simulink model "full_car_model"  (Simulink 7.0)
settings: Solver=ode45  StartTime=0.0  StopTime=120  RelTol=1e-3
undefined symbols (not defined in the file): a, b, c, c01, c02, c03, c04, c1, c2, c3, c4, d, Ix, Iy, k01, k02, k03, k04, k1, k2, k3, k4, M, m1, m2, m3, m4, sigbuilder_block
(part 1 of 2)
settings Model: Creator=Svitlana i Oleksandr  LastModifiedBy=Svitlana i Oleksandr
settings DataIOCC: LimitDataPoints=off

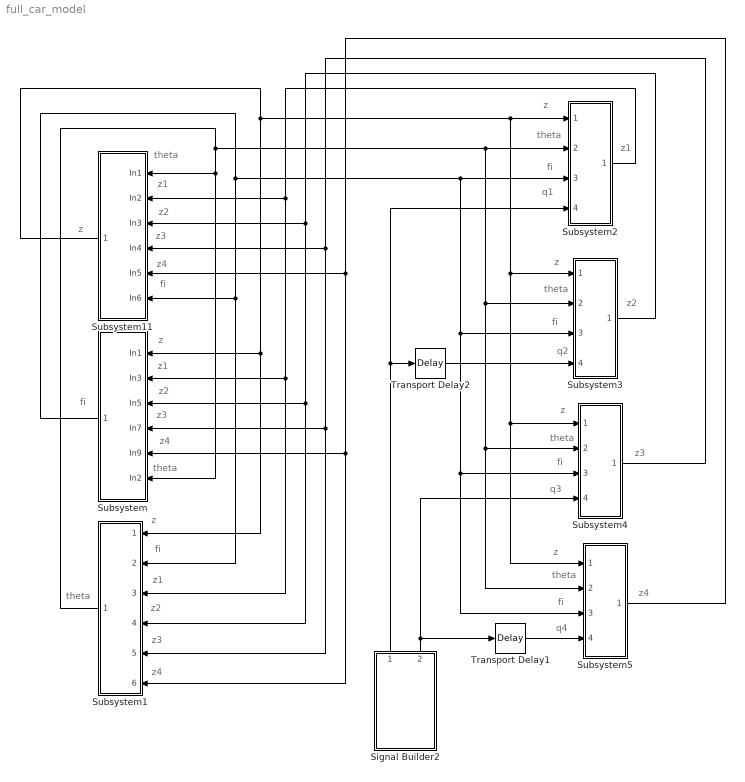
== system full_car_model ==
  note: z
  note: theta
  note: z1
  note: z2
  note: z3
  note: z4
  note: fi
  note: fi
  note: z
  note: z1
  note: z2
  note: z3
  note: z4
  note: theta
  note: theta
  note: z
  note: fi
  note: z1
  note: z2
  note: z3
  note: z4
  note: z1
  note: z
  note: theta
  note: fi
  note: q1
  note: z2
  note: z
  note: theta
  note: fi
  note: q2
  note: z3
  note: z
  note: theta
  note: fi
  note: q3
  note: z4
  note: q4
  note: z
  note: theta
  note: fi
  Signal Builder2 : Subsystem  Tag=STV Subsys  Orientation=up  LoadFcn=sigbuilder_block('load');  StartFcn=sigbuilder_block('start');  StopFcn=sigbuilder_block('stop');  ClipboardFcn=sigbuilder_block('clipboard');  mask(Sigbuilder block){}
      mask help: Sigbuilder GUI
      mask init:
      | if ~strcmp(get_param(bdroot(gcbh),'SimulationStatus'),'stopped') tuvar = sigbuilder_block('maskInit'); end
      settings: CopyFcn=sigbuilder_block('copy');  DeleteFcn=sigbuilder_block('delete');  ModelCloseFcn=sigbuilder_block('modelClose');  PreSaveFcn=sigbuilder_block('preSave');  NameChangeFcn=sigbuilder_block('namechange');  OpenFcn=sigbuilder_block('open',[124.5 96 550.5 363.75 ]);  CloseFcn=sigbuilder_block('close');
      mask Display: plot(0,0,100,100,[10,10,40,40,10],[80,20,20,80,80],[40,10],[50,50], [40,27,10],[65,72,56],[40,25,25,10],[28,28,43,43]);
  Subsystem : Subsystem  Orientation=left
  Subsystem1 : Subsystem  Orientation=left
  Subsystem11 : Subsystem  Orientation=left
  Subsystem2 : Subsystem
  Subsystem3 : Subsystem
  Subsystem4 : Subsystem
  Subsystem5 : Subsystem
  Transport Delay1 : TransportDelay  DelayTime=0.2
  Transport Delay2 : TransportDelay  DelayTime=0.2
  wires:
  Subsystem11/1(Out1) -> Subsystem/1(In1), Subsystem1/1(In1), Subsystem2/1(In1), Subsystem3/1(In1), Subsystem4/1(In1), Subsystem5/1(In1)
  Subsystem/1(Out1) -> Subsystem11/6(In6), Subsystem1/2(In2), Subsystem2/3(In3), Subsystem3/3(In3), Subsystem4/3(In3), Subsystem5/3(In3)
  Subsystem1/1(Out1) -> Subsystem11/1(In1), Subsystem/6(In2), Subsystem2/2(In2), Subsystem3/2(In2), Subsystem4/2(In2), Subsystem5/2(In2)
  Subsystem2/1(Out1) -> Subsystem11/2(In2), Subsystem/2(In3), Subsystem1/3(In3)
  Subsystem3/1(Out1) -> Subsystem11/3(In3), Subsystem/3(In5), Subsystem1/4(In6)
  Transport Delay2/1 -> Subsystem3/4(In4)
  Subsystem4/1(Out1) -> Subsystem11/4(In4), Subsystem/4(In7), Subsystem1/5(In9)
  Subsystem5/1(Out1) -> Subsystem11/5(In5), Subsystem/5(In9), Subsystem1/6(In12)
  Transport Delay1/1 -> Subsystem5/4(In7)
  Signal Builder2/2(Signal 2) -> Transport Delay1/1, Subsystem4/4(In4)
  Signal Builder2/1(Signal 1) -> Subsystem2/4(In4), Transport Delay2/1

== system full_car_model/Signal Builder2 ==
  Demux : Demux  Tag=STV Demux  Outputs=2
  FromWs : FromWorkspace  Tag=STV FromWs  VariableName=tuvar  SampleTime=0  SigBuilderData=DataTag0  VnvData=DataTag1
      SigBuilderData=|
      | channels(1).label = 'Signal 1'
      | channels(1).allXData = {[0 4 4 6 6 10]}
      | channels(1).allYData = {[0 0 0.1 0.1 0 0]}
      | channels(2).label = 'Signal 2'
      | channels(2).allXData = {[0 10]}
      | channels(2).allYData = {[0 0]}
      | common.afterFinalStr = 'Extrapolate'
      | common.sampleTime = 0
      | dataSet.timeRange = [0 10]
      | dataSet.name = 'Group 1'
  Signal 1 : Outport  Tag=STV Outport  OutDataType=sfix(16)  OutScaling=2^0
  Signal 2 : Outport  Tag=STV Outport  Port=2
  wires:
  FromWs/1 -> Demux/1
  Demux/1 -> Signal 1/1
  Demux/2 -> Signal 2/1

== system full_car_model/Subsystem ==
  note: fi
  note: z
  note: theta
  note: fi
  note: z1
  note: k1
  note: c1
  note: k2
  note: c2
  note: z
  note: theta
  note: fi
  note: z2
  note: k3
  note: c3
  note: z
  note: theta
  note: fi
  note: z3
  note: k4
  note: c4
  note: z
  note: theta
  note: fi
  note: z4
  note: fi
  note: theta
  note: z
  In1 : Inport  Orientation=left
  In3 : Inport  Orientation=left  Port=2
  In5 : Inport  Orientation=left  Port=3
  In7 : Inport  Orientation=left  Port=4
  In9 : Inport  Orientation=left  Port=5
  In2 : Inport  Orientation=left  Port=6
  Gain2 : Gain  Gain=1/Ix  ParameterDataType=sfix(16)  ParameterScaling=2^0  OutDataType=sfix(16)  OutScaling=2^0
  Integrator3 : Integrator
  Integrator4 : Integrator
  Subsystem3 : Subsystem  Orientation=left
  Subsystem4 : Subsystem  Orientation=left
  Subsystem5 : Subsystem  Orientation=left
  Subsystem6 : Subsystem  Orientation=left
  Sum2 : Sum  Inputs=----++++  OutDataType=sfix(16)  OutScaling=2^0
  Out1 : Outport
  wires:
  Sum2/1 -> Gain2/1
  Gain2/1 -> Integrator3/1
  Integrator3/1 -> Integrator4/1
  Integrator4/1 -> Subsystem3/3(In3), Subsystem4/3(In3), Subsystem5/3(In3), Subsystem6/3(In3), Out1/1
  Subsystem3/1(Out1) -> Sum2/1
  Subsystem3/2(Out2) -> Sum2/2
  Subsystem4/1(Out1) -> Sum2/3
  Subsystem4/2(Out2) -> Sum2/4
  Subsystem5/1(Out1) -> Sum2/5
  Subsystem5/2(Out2) -> Sum2/6
  Subsystem6/1(Out1) -> Sum2/7
  Subsystem6/2(Out2) -> Sum2/8
  In3/1 -> Subsystem3/4(In4)
  In5/1 -> Subsystem4/4(In4)
  In7/1 -> Subsystem5/4(In4)
  In9/1 -> Subsystem6/4(In4)
  In1/1 -> Subsystem3/1(In1), Subsystem4/1(In1), Subsystem5/1(In1), Subsystem6/1(In1)
  In2/1 -> Subsystem3/2(In2), Subsystem4/2(In2), Subsystem5/2(In2), Subsystem6/2(In2)

== system full_car_model/Subsystem1 ==
  note: theta
  note: k1
  note: c1
  note: z
  note: theta
  note: fi
  note: z1
  note: k2
  note: c2
  note: z
  note: theta
  note: fi
  note: z2
  note: k3
  note: c3
  note: z
  note: theta
  note: fi
  note: z3
  note: k4
  note: c4
  note: z
  note: fi
  note: z
  note: theta
  note: fi
  note: z4
  In1 : Inport  Orientation=left
  In2 : Inport  Orientation=left  Port=2
  In3 : Inport  Orientation=left  Port=3
  In6 : Inport  Orientation=left  Port=4
  In9 : Inport  Orientation=left  Port=5
  In12 : Inport  Orientation=left  Port=6
  Gain3 : Gain  Gain=1/Iy  ParameterDataType=sfix(16)  ParameterScaling=2^0  OutDataType=sfix(16)  OutScaling=2^0
  Integrator5 : Integrator
  Integrator6 : Integrator
  Subsystem10 : Subsystem  Orientation=left
  Subsystem7 : Subsystem  Orientation=left
  Subsystem8 : Subsystem  Orientation=left
  Subsystem9 : Subsystem  Orientation=left
  Sum3 : Sum  Inputs=++--++--  OutDataType=sfix(16)  OutScaling=2^0
  Out1 : Outport
  wires:
  Sum3/1 -> Gain3/1
  Gain3/1 -> Integrator5/1
  Integrator5/1 -> Integrator6/1
  Subsystem7/1(Out1) -> Sum3/1
  Subsystem7/2(Out2) -> Sum3/2
  Subsystem8/1(Out1) -> Sum3/3
  Subsystem8/2(Out2) -> Sum3/4
  Subsystem9/1(Out1) -> Sum3/5
  Subsystem9/2(Out2) -> Sum3/6
  Subsystem10/1(Out1) -> Sum3/7
  Subsystem10/2(Out2) -> Sum3/8
  Integrator6/1 -> Subsystem7/2(In2), Subsystem8/2(In2), Subsystem9/2(In2), Subsystem10/2(In2), Out1/1
  In3/1 -> Subsystem7/4(In4)
  In6/1 -> Subsystem8/4(In4)
  In9/1 -> Subsystem9/4(In4)
  In12/1 -> Subsystem10/4(In4)
  In1/1 -> Subsystem7/1(In1), Subsystem8/1(In1), Subsystem9/1(In1), Subsystem10/1(In1)
  In2/1 -> Subsystem7/3(In3), Subsystem8/3(In3), Subsystem9/3(In3), Subsystem10/3(In3)

== system full_car_model/Subsystem11 ==
  note: z
  note: z
  note: theta
  note: fi
  note: z1
  note: k1
  note: c1
  note: z
  note: theta
  note: fi
  note: z2
  note: k2
  note: c2
  note: z
  note: theta
  note: fi
  note: z3
  note: k3
  note: c3
  note: z
  note: theta
  note: fi
  note: z4
  note: z
  note: theta
  note: k4
  note: c4
  note: fi
  In1 : Inport  Orientation=left  OutDataType=sfix(16)  OutScaling=2^0
  In2 : Inport  Orientation=left  Port=2  OutDataType=sfix(16)  OutScaling=2^0
  In3 : Inport  Orientation=left  Port=3  OutDataType=sfix(16)  OutScaling=2^0
  In4 : Inport  Orientation=left  Port=4  OutDataType=sfix(16)  OutScaling=2^0
  In5 : Inport  Orientation=left  Port=5  OutDataType=sfix(16)  OutScaling=2^0
  In6 : Inport  Orientation=left  Port=6  OutDataType=sfix(16)  OutScaling=2^0
  Gain1 : Gain  Gain=1/M  ParameterDataType=sfix(16)  ParameterScaling=2^0  OutDataType=sfix(16)  OutScaling=2^0
  Integrator1 : Integrator
  Integrator2 : Integrator
  Subsystem : Subsystem  Orientation=left
  Subsystem1 : Subsystem  Orientation=left
  Subsystem2 : Subsystem  Orientation=left
  Subsystem40 : Subsystem  Orientation=left
  Sum1 : Sum  Inputs=--------  OutDataType=sfix(16)  OutScaling=2^0
  Out1 : Outport  OutDataType=sfix(16)  OutScaling=2^0
  wires:
  Sum1/1 -> Gain1/1
  Gain1/1 -> Integrator1/1
  Integrator1/1 -> Integrator2/1
  Subsystem40/1(Out1) -> Sum1/8
  Subsystem40/2(Out2) -> Sum1/7
  Subsystem/1(Out1) -> Sum1/6
  Subsystem/2(Out2) -> Sum1/5
  In2/1 -> Subsystem40/4(In4)
  In3/1 -> Subsystem/4(In4)
  In4/1 -> Subsystem1/4(In4)
  In5/1 -> Subsystem2/4(In4)
  Integrator2/1 -> Out1/1, Subsystem40/1(In1), Subsystem/1(In1), Subsystem1/1(In1), Subsystem2/1(In1)
  Subsystem1/1(Out1) -> Sum1/4
  Subsystem1/2(Out2) -> Sum1/3
  Subsystem2/1(Out1) -> Sum1/2
  Subsystem2/2(Out2) -> Sum1/1
  In1/1 -> Subsystem40/2(In2), Subsystem/2(In2), Subsystem1/2(In2), Subsystem2/2(In2)
  In6/1 -> Subsystem40/3(In3), Subsystem/3(In3), Subsystem1/3(In3), Subsystem2/3(In3)

== system full_car_model/Subsystem2 ==
  note: z1
  note: k1
  note: z
  note: theta
  note: fi
  note: z1
  note: c1
  note: z
  note: theta
  note: fi
  note: z1
  note: k01
  note: z1
  note: q1
  note: c01
  note: z1
  note: q1
  note: z
  note: theta
  note: fi
  note: q1
  In1 : Inport  Orientation=left
  In2 : Inport  Orientation=left  Port=2
  In3 : Inport  Orientation=left  Port=3
  In4 : Inport  Orientation=left  Port=4
  Gain4 : Gain  Gain=1/m1  ParameterDataType=sfix(16)  ParameterScaling=2^0  OutDataType=sfix(16)  OutScaling=2^0
  Integrator7 : Integrator
  Integrator8 : Integrator
  Subsystem24 : Subsystem  Orientation=left
  Subsystem25 : Subsystem  Orientation=left
  Subsystem26 : Subsystem  Orientation=left
  Subsystem27 : Subsystem  Orientation=left
  Sum8 : Sum  Inputs=++--  OutDataType=sfix(16)  OutScaling=2^0
  Out1 : Outport  OutDataType=sfix(16)  OutScaling=2^0
  wires:
  Gain4/1 -> Integrator7/1
  Integrator7/1 -> Integrator8/1
  Sum8/1 -> Gain4/1
  Subsystem24/1(Out2) -> Sum8/1
  Subsystem25/1(Out2) -> Sum8/2
  Subsystem26/1(Out2) -> Sum8/3
  Subsystem27/1(Out2) -> Sum8/4
  In1/1 -> Subsystem24/1(In1), Subsystem25/1(In1)
  In2/1 -> Subsystem24/2(In3), Subsystem25/2(In3)
  In3/1 -> Subsystem24/3(In4), Subsystem25/3(In4)
  Integrator8/1 -> Out1/1, Subsystem24/4(In5), Subsystem25/4(In5), Subsystem26/1(In1), Subsystem27/1(In1)
  In4/1 -> Subsystem26/2(In5), Subsystem27/2(In5)

== system full_car_model/Subsystem3 ==
  note: z2
  note: k2
  note: z
  note: theta
  note: fi
  note: z2
  note: c2
  note: z
  note: theta
  note: fi
  note: z2
  note: k02
  note: z2
  note: q2
  note: c02
  note: z2
  note: q2
  note: z
  note: fi
  note: q2
  In1 : Inport  Orientation=left
  In2 : Inport  Orientation=left  Port=2
  In3 : Inport  Orientation=left  Port=3
  In4 : Inport  Orientation=left  Port=4
  Gain5 : Gain  Gain=1/m2  ParameterDataType=sfix(16)  ParameterScaling=2^0  OutDataType=sfix(16)  OutScaling=2^0
  Integrator10 : Integrator
  Integrator9 : Integrator
  Subsystem28 : Subsystem  Orientation=left
  Subsystem29 : Subsystem  Orientation=left
  Subsystem30 : Subsystem  Orientation=left
  Subsystem31 : Subsystem  Orientation=left
  Sum5 : Sum  Inputs=++--  OutDataType=sfix(16)  OutScaling=2^0
  Out1 : Outport  OutDataType=sfix(16)  OutScaling=2^0
  wires:
  Sum5/1 -> Gain5/1
  Gain5/1 -> Integrator9/1
  Integrator9/1 -> Integrator10/1
  Subsystem28/1(Out2) -> Sum5/1
  Subsystem29/1(Out2) -> Sum5/2
  Subsystem30/1(Out2) -> Sum5/3
  Subsystem31/1(Out2) -> Sum5/4
  In1/1 -> Subsystem28/1(In1), Subsystem29/1(In1)
  In2/1 -> Subsystem28/2(In3), Subsystem29/2(In3)
  In3/1 -> Subsystem28/3(In4), Subsystem29/3(In4)
  Integrator10/1 -> Out1/1, Subsystem28/4(In5), Subsystem29/4(In5), Subsystem30/1(In1), Subsystem31/1(In1)
  In4/1 -> Subsystem30/2(In5), Subsystem31/2(In5)

== system full_car_model/Subsystem4 ==
  note: z3
  note: c3
  note: z
  note: theta
  note: fi
  note: z3
  note: k3
  note: z
  note: theta
  note: fi
  note: z3
  note: k03
  note: z3
  note: q3
  note: c03
  note: z3
  note: q3
  note: z
  note: theta
  note: fi
  note: q3
  In1 : Inport  Orientation=left
  In2 : Inport  Orientation=left  Port=2
  In3 : Inport  Orientation=left  Port=3
  In4 : Inport  Orientation=left  Port=4
  Gain6 : Gain  Gain=1/m3  ParameterDataType=sfix(16)  ParameterScaling=2^0  OutDataType=sfix(16)  OutScaling=2^0
  Integrator11 : Integrator
  Integrator12 : Integrator
  Subsystem32 : Subsystem  Orientation=left
  Subsystem33 : Subsystem  Orientation=left
  Subsystem34 : Subsystem  Orientation=left
  Subsystem35 : Subsystem  Orientation=left
  Sum6 : Sum  Inputs=++--  OutDataType=sfix(16)  OutScaling=2^0
  Out1 : Outport  OutDataType=sfix(16)  OutScaling=2^0
  wires:
  Sum6/1 -> Gain6/1
  Gain6/1 -> Integrator12/1
  Integrator12/1 -> Integrator11/1
  Subsystem32/1(Out2) -> Sum6/1
  Subsystem33/1(Out2) -> Sum6/2
  Subsystem34/1(Out2) -> Sum6/3
  Subsystem35/1(Out2) -> Sum6/4
  In1/1 -> Subsystem32/1(In1), Subsystem33/1(In1)
  In2/1 -> Subsystem32/2(In3), Subsystem33/2(In3)
  In3/1 -> Subsystem32/3(In4), Subsystem33/3(In4)
  Integrator11/1 -> Out1/1, Subsystem32/4(In5), Subsystem33/4(In5), Subsystem34/1(In1), Subsystem35/1(In1)
  In4/1 -> Subsystem34/2(In5), Subsystem35/2(In5)

== system full_car_model/Subsystem5 ==
  note: z4
  note: k4
  note: z
  note: theta
  note: fi
  note: z4
  note: c4
  note: z
  note: theta
  note: fi
  note: z4
  note: k04
  note: z4
  note: q4
  note: c04
  note: z4
  note: q4
  note: z
  note: theta
  note: fi
  note: z4
  note: q4
  In1 : Inport  Orientation=left
  In2 : Inport  Orientation=left  Port=2
  In3 : Inport  Orientation=left  Port=3
  In7 : Inport  Orientation=left  Port=4
  Gain7 : Gain  Gain=1/m4  ParameterDataType=sfix(16)  ParameterScaling=2^0  OutDataType=sfix(16)  OutScaling=2^0
  Integrator13 : Integrator
  Integrator14 : Integrator
  Subsystem36 : Subsystem  Orientation=left
  Subsystem37 : Subsystem  Orientation=left
  Subsystem38 : Subsystem  Orientation=left
  Subsystem39 : Subsystem  Orientation=left
  Sum7 : Sum  Inputs=++--  OutDataType=sfix(16)  OutScaling=2^0
  Out1 : Outport  OutDataType=sfix(16)  OutScaling=2^0
  wires:
  Sum7/1 -> Gain7/1
  Gain7/1 -> Integrator14/1
  Integrator14/1 -> Integrator13/1
  Subsystem36/1(Out2) -> Sum7/1
  Subsystem37/1(Out2) -> Sum7/2
  Subsystem38/1(Out2) -> Sum7/3
  Subsystem39/1(Out2) -> Sum7/4
  In1/1 -> Subsystem36/1(In1), Subsystem37/1(In1)
  In2/1 -> Subsystem36/2(In3), Subsystem37/2(In3)
  In3/1 -> Subsystem36/3(In4), Subsystem37/3(In4)
  In7/1 -> Subsystem38/2(In5), Subsystem39/2(In5)
  Integrator13/1 -> Out1/1, Subsystem36/4(In5), Subsystem37/4(In5), Subsystem38/1(In1), Subsystem39/1(In1)

== system full_car_model/Subsystem/Subsystem3 ==
  note: z
  note: k1
  note: theta
  note: fi
  note: z1
  note: c1
  note: z
  note: theta
  note: fi
  note: z1
  note: z
  note: theta
  note: fi
  note: z1
  In1 : Inport  Orientation=left
  In2 : Inport  Orientation=left  Port=2
  In3 : Inport  Orientation=left  Port=3
  In4 : Inport  Orientation=left  Port=4
  Constant1 : Constant  Orientation=left  Value=c  OutDataType=sfix(16)  OutScaling=2^0
  Constant2 : Constant  Orientation=left  Value=c  OutDataType=sfix(16)  OutScaling=2^0
  Product2 : Product  Orientation=left  OutDataType=sfix(16)  OutScaling=2^0  RndMeth=Zero
  Product3 : Product  Orientation=left  OutDataType=sfix(16)  OutScaling=2^0  RndMeth=Zero
  Subsystem8 : Subsystem  Orientation=left
  Subsystem9 : Subsystem  Orientation=left
  Out1 : Outport  Orientation=left
  Out2 : Outport  Orientation=left  Port=2
  wires:
  Subsystem8/1(Out2) -> Product2/1
  Constant1/1 -> Product2/2
  Subsystem9/1(Out2) -> Product3/1
  Constant2/1 -> Product3/2
  In1/1 -> Subsystem8/1(In1), Subsystem9/1(In1)
  In2/1 -> Subsystem8/2(In3), Subsystem9/2(In3)
  In3/1 -> Subsystem8/3(In4), Subsystem9/3(In4)
  Product2/1 -> Out1/1
  Product3/1 -> Out2/1
  In4/1 -> Subsystem8/4(In5), Subsystem9/4(In5)

== system full_car_model/Subsystem/Subsystem4 ==
  note: k2
  note: z
  note: theta
  note: fi
  note: z2
  note: c2
  note: z
  note: theta
  note: fi
  note: z2
  note: z
  note: theta
  note: fi
  note: z2
  In1 : Inport  Orientation=left
  In2 : Inport  Orientation=left  Port=2
  In3 : Inport  Orientation=left  Port=3
  In4 : Inport  Orientation=left  Port=4
  Constant3 : Constant  Orientation=left  Value=c  OutDataType=sfix(16)  OutScaling=2^0
  Constant4 : Constant  Orientation=left  Value=c  OutDataType=sfix(16)  OutScaling=2^0
  Product4 : Product  Orientation=left  OutDataType=sfix(16)  OutScaling=2^0  RndMeth=Zero
  Product5 : Product  Orientation=left  OutDataType=sfix(16)  OutScaling=2^0  RndMeth=Zero
  Subsystem10 : Subsystem  Orientation=left
  Subsystem11 : Subsystem  Orientation=left
  Out1 : Outport  Orientation=left
  Out2 : Outport  Orientation=left  Port=2
  wires:
  Subsystem10/1(Out2) -> Product4/1
  Constant3/1 -> Product4/2
  Subsystem11/1(Out2) -> Product5/1
  Constant4/1 -> Product5/2
  In1/1 -> Subsystem10/1(In1), Subsystem11/1(In1)
  In2/1 -> Subsystem10/2(In3), Subsystem11/2(In3)
  In3/1 -> Subsystem10/3(In4), Subsystem11/3(In4)
  Product4/1 -> Out1/1
  Product5/1 -> Out2/1
  In4/1 -> Subsystem10/4(In5), Subsystem11/4(In5)

== system full_car_model/Subsystem/Subsystem5 ==
  note: k3
  note: z
  note: theta
  note: fi
  note: z3
  note: c3
  note: z
  note: theta
  note: fi
  note: z3
  note: z
  note: theta
  note: fi
  note: z3
  In1 : Inport  Orientation=left
  In2 : Inport  Orientation=left  Port=2
  In3 : Inport  Orientation=left  Port=3
  In4 : Inport  Orientation=left  Port=4
  Constant5 : Constant  Orientation=left  Value=d  OutDataType=sfix(16)  OutScaling=2^0
  Constant6 : Constant  Orientation=left  Value=d  OutDataType=sfix(16)  OutScaling=2^0
  Product6 : Product  Orientation=left  OutDataType=sfix(16)  OutScaling=2^0  RndMeth=Zero
  Product7 : Product  Orientation=left  OutDataType=sfix(16)  OutScaling=2^0  RndMeth=Zero
  Subsystem12 : Subsystem  Orientation=left
  Subsystem13 : Subsystem  Orientation=left
  Out1 : Outport  Orientation=left
  Out2 : Outport  Orientation=left  Port=2
  wires:
  Subsystem12/1(Out2) -> Product6/1
  Constant5/1 -> Product6/2
  Subsystem13/1(Out2) -> Product7/1
  Constant6/1 -> Product7/2
  In1/1 -> Subsystem12/1(In1), Subsystem13/1(In1)
  In2/1 -> Subsystem12/2(In3), Subsystem13/2(In3)
  In3/1 -> Subsystem12/3(In4), Subsystem13/3(In4)
  Product6/1 -> Out1/1
  Product7/1 -> Out2/1
  In4/1 -> Subsystem12/4(In5), Subsystem13/4(In5)

== system full_car_model/Subsystem/Subsystem6 ==
  note: k4
  note: z
  note: theta
  note: fi
  note: z4
  note: c4
  note: z
  note: theta
  note: fi
  note: z4
  note: z
  note: theta
  note: z4
  note: fi
  In1 : Inport  Orientation=down
  In2 : Inport  Orientation=down  Port=2
  In3 : Inport  Orientation=down  Port=3
  In4 : Inport  Orientation=down  Port=4
  Constant7 : Constant  Orientation=left  Value=d  OutDataType=sfix(16)  OutScaling=2^0
  Constant8 : Constant  Orientation=left  Value=d  OutDataType=sfix(16)  OutScaling=2^0
  Product8 : Product  Orientation=left  OutDataType=sfix(16)  OutScaling=2^0  RndMeth=Zero
  Product9 : Product  Orientation=left  OutDataType=sfix(16)  OutScaling=2^0  RndMeth=Zero
  Subsystem14 : Subsystem  Orientation=left
  Subsystem15 : Subsystem  Orientation=left
  Out1 : Outport  Orientation=left
  Out2 : Outport  Orientation=left  Port=2
  wires:
  Subsystem14/1(Out2) -> Product8/1
  Constant7/1 -> Product8/2
  Subsystem15/1(Out2) -> Product9/1
  Constant8/1 -> Product9/2
  In1/1 -> Subsystem14/1(In1), Subsystem15/1(In1)
  In2/1 -> Subsystem14/2(In3), Subsystem15/2(In3)
  In3/1 -> Subsystem14/3(In4), Subsystem15/3(In4)
  In4/1 -> Subsystem14/4(In5), Subsystem15/4(In5)
  Product8/1 -> Out1/1
  Product9/1 -> Out2/1

== system full_car_model/Subsystem1/Subsystem10 ==
  note: k4
  note: z
  note: theta
  note: fi
  note: z4
  note: c4
  note: z
  note: theta
  note: fi
  note: z4
  In1 : Inport  Orientation=down
  In2 : Inport  Orientation=down  Port=2
  In3 : Inport  Orientation=down  Port=3
  In4 : Inport  Orientation=down  Port=4
  Constant15 : Constant  Orientation=left  Value=b  OutDataType=sfix(16)  OutScaling=2^0
  Constant16 : Constant  Orientation=left  Value=b  OutDataType=sfix(16)  OutScaling=2^0
  Product16 : Product  Orientation=left  OutDataType=sfix(16)  OutScaling=2^0  RndMeth=Zero
  Product17 : Product  Orientation=left  OutDataType=sfix(16)  OutScaling=2^0  RndMeth=Zero
  Subsystem20 : Subsystem  Orientation=left
  Subsystem21 : Subsystem  Orientation=left
  Out1 : Outport  Orientation=left
  Out2 : Outport  Orientation=left  Port=2
  wires:
  Subsystem20/1(Out2) -> Product16/1
  Constant15/1 -> Product16/2
  Subsystem21/1(Out2) -> Product17/1
  Constant16/1 -> Product17/2
  In1/1 -> Subsystem20/1(In1), Subsystem21/1(In1)
  In2/1 -> Subsystem20/2(In3), Subsystem21/2(In3)
  In3/1 -> Subsystem20/3(In4), Subsystem21/3(In4)
  In4/1 -> Subsystem20/4(In5), Subsystem21/4(In5)
  Product16/1 -> Out1/1
  Product17/1 -> Out2/1

== system full_car_model/Subsystem1/Subsystem7 ==
  note: z
  note: k1
  note: theta
  note: fi
  note: z1
  note: c1
  note: z
  note: theta
  note: fi
  note: z1
  note: z
  note: theta
  note: fi
  note: z1
  In1 : Inport  Orientation=left
  In2 : Inport  Orientation=left  Port=2
  In3 : Inport  Orientation=left  Port=3
  In4 : Inport  Orientation=left  Port=4
  Constant10 : Constant  Orientation=left  Value=a  OutDataType=sfix(16)  OutScaling=2^0
  Constant9 : Constant  Orientation=left  Value=a  OutDataType=sfix(16)  OutScaling=2^0
  Product10 : Product  Orientation=left  OutDataType=sfix(16)  OutScaling=2^0  RndMeth=Zero
  Product11 : Product  Orientation=left  OutDataType=sfix(16)  OutScaling=2^0  RndMeth=Zero
  Subsystem22 : Subsystem  Orientation=left
  Subsystem23 : Subsystem  Orientation=left
  Out1 : Outport  Orientation=left
  Out2 : Outport  Orientation=left  Port=2
  wires:
  Subsystem22/1(Out2) -> Product10/1
  Constant9/1 -> Product10/2
  Subsystem23/1(Out2) -> Product11/1
  Constant10/1 -> Product11/2
  In1/1 -> Subsystem22/1(In1), Subsystem23/1(In1)
  In2/1 -> Subsystem22/2(In3), Subsystem23/2(In3)
  In3/1 -> Subsystem22/3(In4), Subsystem23/3(In4)
  Product10/1 -> Out1/1
  Product11/1 -> Out2/1
  In4/1 -> Subsystem22/4(In5), Subsystem23/4(In5)

== system full_car_model/Subsystem1/Subsystem8 ==
  note: k2
  note: z
  note: theta
  note: fi
  note: z2
  note: c2
  note: z
  note: theta
  note: fi
  note: z2
  note: z
  note: theta
  note: fi
  note: z2
  In1 : Inport  Orientation=left
  In2 : Inport  Orientation=left  Port=2
  In3 : Inport  Orientation=left  Port=3
  In4 : Inport  Orientation=left  Port=4
  Constant11 : Constant  Orientation=left  Value=b  OutDataType=sfix(16)  OutScaling=2^0
  Constant12 : Constant  Orientation=left  Value=b  OutDataType=sfix(16)  OutScaling=2^0
  Product12 : Product  Orientation=left  OutDataType=sfix(16)  OutScaling=2^0  RndMeth=Zero
  Product13 : Product  Orientation=left  OutDataType=sfix(16)  OutScaling=2^0  RndMeth=Zero
  Subsystem16 : Subsystem  Orientation=left
  Subsystem17 : Subsystem  Orientation=left
  Out1 : Outport  Orientation=left
  Out2 : Outport  Orientation=left  Port=2
  wires:
  Subsystem16/1(Out2) -> Product12/1
  Constant11/1 -> Product12/2
  Subsystem17/1(Out2) -> Product13/1
  Constant12/1 -> Product13/2
  In1/1 -> Subsystem16/1(In1), Subsystem17/1(In1)
  In2/1 -> Subsystem16/2(In3), Subsystem17/2(In3)
  In3/1 -> Subsystem16/3(In4), Subsystem17/3(In4)
  Product12/1 -> Out1/1
  Product13/1 -> Out2/1
  In4/1 -> Subsystem16/4(In5), Subsystem17/4(In5)

== system full_car_model/Subsystem1/Subsystem9 ==
  note: k3
  note: z
  note: theta
  note: fi
  note: z3
  note: c3
  note: z
  note: theta
  note: fi
  note: z3
  note: z
  note: theta
  note: fi
  note: z3
  In1 : Inport  Orientation=left
  In2 : Inport  Orientation=left  Port=2
  In3 : Inport  Orientation=left  Port=3
  In4 : Inport  Orientation=left  Port=4
  Constant13 : Constant  Orientation=left  Value=a  OutDataType=sfix(16)  OutScaling=2^0
  Constant14 : Constant  Orientation=left  Value=a  OutDataType=sfix(16)  OutScaling=2^0
  Product14 : Product  Orientation=left  OutDataType=sfix(16)  OutScaling=2^0  RndMeth=Zero
  Product15 : Product  Orientation=left  OutDataType=sfix(16)  OutScaling=2^0  RndMeth=Zero
  Subsystem18 : Subsystem  Orientation=left
  Subsystem19 : Subsystem  Orientation=left
  Out1 : Outport  Orientation=left
  Out2 : Outport  Orientation=left  Port=2
  wires:
  Subsystem18/1(Out2) -> Product14/1
  Constant13/1 -> Product14/2
  Subsystem19/1(Out2) -> Product15/1
  Constant14/1 -> Product15/2
  In1/1 -> Subsystem18/1(In1), Subsystem19/1(In1)
  In2/1 -> Subsystem18/2(In3), Subsystem19/2(In3)
  In3/1 -> Subsystem18/3(In4), Subsystem19/3(In4)
  Product14/1 -> Out1/1
  Product15/1 -> Out2/1
  In4/1 -> Subsystem18/4(In5), Subsystem19/4(In5)

== system full_car_model/Subsystem11/Subsystem ==
  note: k2
  note: theta
  note: fi
  note: z2
  note: c2
  note: z
  note: theta
  note: fi
  note: z2
  note: z
  note: z
  note: theta
  note: fi
  note: z2
  In1 : Inport  Orientation=left
  In2 : Inport  Orientation=left  Port=2
  In3 : Inport  Orientation=left  Port=3
  In4 : Inport  Orientation=left  Port=4
  Subsystem2 : Subsystem  Orientation=left
  Subsystem3 : Subsystem  Orientation=left
  Out1 : Outport  Orientation=left
  Out2 : Outport  Orientation=left  Port=2
  wires:
  In1/1 -> Subsystem2/1(In1), Subsystem3/1(In1)
  In2/1 -> Subsystem2/2(In3), Subsystem3/2(In3)
  In3/1 -> Subsystem2/3(In4), Subsystem3/3(In4)
  Subsystem2/1(Out2) -> Out1/1
  Subsystem3/1(Out2) -> Out2/1
  In4/1 -> Subsystem2/4(In5), Subsystem3/4(In5)

== system full_car_model/Subsystem11/Subsystem1 ==
  note: k3
  note: z
  note: theta
  note: fi
  note: z3
  note: c3
  note: z
  note: theta
  note: fi
  note: z3
  note: z
  note: theta
  note: fi
  note: z3
  In1 : Inport  Orientation=left
  In2 : Inport  Orientation=left  Port=2
  In3 : Inport  Orientation=left  Port=3
  In4 : Inport  Orientation=left  Port=4
  Subsystem4 : Subsystem  Orientation=left
  Subsystem5 : Subsystem  Orientation=left
  Out1 : Outport  Orientation=left
  Out2 : Outport  Orientation=left  Port=2
  wires:
  In1/1 -> Subsystem4/1(In1), Subsystem5/1(In1)
  In2/1 -> Subsystem4/2(In3), Subsystem5/2(In3)
  In3/1 -> Subsystem4/3(In4), Subsystem5/3(In4)
  Subsystem4/1(Out2) -> Out1/1
  Subsystem5/1(Out2) -> Out2/1
  In4/1 -> Subsystem4/4(In5), Subsystem5/4(In5)

== system full_car_model/Subsystem11/Subsystem2 ==
  note: k4
  note: z
  note: theta
  note: fi
  note: z4
  note: c4
  note: z
  note: theta
  note: fi
  note: z4
  In1 : Inport  Orientation=down
  In2 : Inport  Orientation=down  Port=2
  In3 : Inport  Orientation=down  Port=3
  In4 : Inport  Orientation=down  Port=4
  Subsystem6 : Subsystem  Orientation=left
  Subsystem7 : Subsystem  Orientation=left
  Out1 : Outport  Orientation=left
  Out2 : Outport  Orientation=left  Port=2
  wires:
  In1/1 -> Subsystem6/1(In1), Subsystem7/1(In1)
  In2/1 -> Subsystem6/2(In3), Subsystem7/2(In3)
  In3/1 -> Subsystem6/3(In4), Subsystem7/3(In4)
  In4/1 -> Subsystem6/4(In5), Subsystem7/4(In5)
  Subsystem6/1(Out2) -> Out1/1
  Subsystem7/1(Out2) -> Out2/1

== system full_car_model/Subsystem11/Subsystem40 ==
  note: k1
  note: z
  note: theta
  note: fi
  note: z1
  note: z
  note: theta
  note: fi
  note: z1
  note: c1
  note: z1
  note: z
  note: theta
  note: fi
  In1 : Inport  Orientation=left
  In2 : Inport  Orientation=left  Port=2
  In3 : Inport  Orientation=left  Port=3
  In4 : Inport  Orientation=left  Port=4
  Subsystem : Subsystem  Orientation=left
  Subsystem1 : Subsystem  Orientation=left
  Out1 : Outport  Orientation=left
  Out2 : Outport  Orientation=left  Port=2
  wires:
  In1/1 -> Subsystem/1(In1), Subsystem1/1(In1)
  In2/1 -> Subsystem/2(In3), Subsystem1/2(In3)
  In3/1 -> Subsystem/3(In4), Subsystem1/3(In4)
  In4/1 -> Subsystem/4(In5), Subsystem1/4(In5)
  Subsystem/1(Out2) -> Out1/1
  Subsystem1/1(Out2) -> Out2/1

== system full_car_model/Subsystem2/Subsystem24 ==
  note: z
  note: theta
  note: fi
  note: z1
  In1 : Inport  OutDataType=sfix(16)  OutScaling=2^0
  In3 : Inport  Port=2  OutDataType=sfix(16)  OutScaling=2^0
  In4 : Inport  Port=3  OutDataType=sfix(16)  OutScaling=2^0
  In5 : Inport  Port=4  OutDataType=sfix(16)  OutScaling=2^0
  Constant1 : Constant  Value=a  OutDataType=sfix(16)  OutScaling=2^0
  Constant2 : Constant  Value=c  OutDataType=sfix(16)  OutScaling=2^0
  Gain1 : Gain  Gain=k1  ParameterDataType=sfix(16)  ParameterScaling=2^0  OutDataType=sfix(16)  OutScaling=2^0
  Product1 : Product  OutDataType=sfix(16)  OutScaling=2^0  RndMeth=Zero
  Product2 : Product  OutDataType=sfix(16)  OutScaling=2^0  RndMeth=Zero
  Sum1 : Sum  Inputs=+-+  OutDataType=sfix(16)  OutScaling=2^0
  Sum2 : Sum  Inputs=+-  OutDataType=sfix(16)  OutScaling=2^0
  Out2 : Outport  OutDataType=sfix(16)  OutScaling=2^0
  wires:
  In1/1 -> Sum1/1
  In3/1 -> Product1/1
  In4/1 -> Product2/1
  Constant1/1 -> Product1/2
  Product1/1 -> Sum1/2
  Constant2/1 -> Product2/2
  Product2/1 -> Sum1/3
  Gain1/1 -> Out2/1
  Sum1/1 -> Sum2/1
  In5/1 -> Sum2/2
  Sum2/1 -> Gain1/1

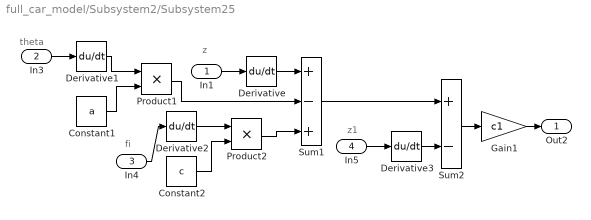
== system full_car_model/Subsystem2/Subsystem25 ==
  note: z1
  note: fi
  note: theta
  note: z
  In1 : Inport  OutDataType=sfix(16)  OutScaling=2^0
  In3 : Inport  Port=2  OutDataType=sfix(16)  OutScaling=2^0
  In4 : Inport  Port=3  OutDataType=sfix(16)  OutScaling=2^0
  In5 : Inport  Port=4  OutDataType=sfix(16)  OutScaling=2^0
  Constant1 : Constant  Value=a  OutDataType=sfix(16)  OutScaling=2^0
  Constant2 : Constant  Value=c  OutDataType=sfix(16)  OutScaling=2^0
  Derivative{,1..3} (4 alike) : Derivative
  Gain1 : Gain  Gain=c1  ParameterDataType=sfix(16)  ParameterScaling=2^0  OutDataType=sfix(16)  OutScaling=2^0
  Product1 : Product  OutDataType=sfix(16)  OutScaling=2^0  RndMeth=Zero
  Product2 : Product  OutDataType=sfix(16)  OutScaling=2^0  RndMeth=Zero
  Sum1 : Sum  Inputs=+-+  OutDataType=sfix(16)  OutScaling=2^0
  Sum2 : Sum  Inputs=+-  OutDataType=sfix(16)  OutScaling=2^0
  Out2 : Outport  OutDataType=sfix(16)  OutScaling=2^0
  wires:
  Gain1/1 -> Out2/1
  Product2/1 -> Sum1/3
  In5/1 -> Derivative3/1
  Constant2/1 -> Product2/2
  Product1/1 -> Sum1/2
  Constant1/1 -> Product1/2
  In4/1 -> Derivative2/1
  In3/1 -> Derivative1/1
  In1/1 -> Derivative/1
  Derivative/1 -> Sum1/1
  Derivative1/1 -> Product1/1
  Derivative2/1 -> Product2/1
  Sum1/1 -> Sum2/1
  Derivative3/1 -> Sum2/2
  Sum2/1 -> Gain1/1

== system full_car_model/Subsystem2/Subsystem26 ==
  note: q1
  note: z1
  In1 : Inport  OutDataType=sfix(16)  OutScaling=2^0
  In5 : Inport  Port=2  OutDataType=sfix(16)  OutScaling=2^0
  Gain1 : Gain  Gain=k01  ParameterDataType=sfix(16)  ParameterScaling=2^0  OutDataType=sfix(16)  OutScaling=2^0
  Sum1 : Sum  Inputs=+-  OutDataType=sfix(16)  OutScaling=2^0
  Out2 : Outport  OutDataType=sfix(16)  OutScaling=2^0
  wires:
  Gain1/1 -> Out2/1
  Sum1/1 -> Gain1/1
  In1/1 -> Sum1/1
  In5/1 -> Sum1/2

== system full_car_model/Subsystem2/Subsystem27 ==
  note: z1
  note: q1
  In1 : Inport  OutDataType=sfix(16)  OutScaling=2^0
  In5 : Inport  Port=2  OutDataType=sfix(16)  OutScaling=2^0
  Derivative : Derivative
  Derivative1 : Derivative
  Gain1 : Gain  Gain=c01  ParameterDataType=sfix(16)  ParameterScaling=2^0  OutDataType=sfix(16)  OutScaling=2^0
  Sum1 : Sum  Inputs=+-  OutDataType=sfix(16)  OutScaling=2^0
  Out2 : Outport  OutDataType=sfix(16)  OutScaling=2^0
  wires:
  In5/1 -> Derivative1/1
  In1/1 -> Derivative/1
  Sum1/1 -> Gain1/1
  Gain1/1 -> Out2/1
  Derivative/1 -> Sum1/1
  Derivative1/1 -> Sum1/2

== system full_car_model/Subsystem3/Subsystem28 ==
  note: z2
  note: fi
  note: theta
  note: z
  In1 : Inport  OutDataType=sfix(16)  OutScaling=2^0
  In3 : Inport  Port=2  OutDataType=sfix(16)  OutScaling=2^0
  In4 : Inport  Port=3  OutDataType=sfix(16)  OutScaling=2^0
  In5 : Inport  Port=4  OutDataType=sfix(16)  OutScaling=2^0
  Constant1 : Constant  Value=b  OutDataType=sfix(16)  OutScaling=2^0
  Constant2 : Constant  Value=c  OutDataType=sfix(16)  OutScaling=2^0
  Gain1 : Gain  Gain=k2  ParameterDataType=sfix(16)  ParameterScaling=2^0  OutDataType=sfix(16)  OutScaling=2^0
  Product1 : Product  OutDataType=sfix(16)  OutScaling=2^0  RndMeth=Zero
  Product2 : Product  OutDataType=sfix(16)  OutScaling=2^0  RndMeth=Zero
  Sum1 : Sum  Inputs=+++  OutDataType=sfix(16)  OutScaling=2^0
  Sum2 : Sum  Inputs=+-  OutDataType=sfix(16)  OutScaling=2^0
  Out2 : Outport  OutDataType=sfix(16)  OutScaling=2^0
  wires:
  Gain1/1 -> Out2/1
  Product2/1 -> Sum1/3
  Constant2/1 -> Product2/2
  Product1/1 -> Sum1/2
  Constant1/1 -> Product1/2
  In4/1 -> Product2/1
  In3/1 -> Product1/1
  In1/1 -> Sum1/1
  Sum1/1 -> Sum2/1
  In5/1 -> Sum2/2
  Sum2/1 -> Gain1/1

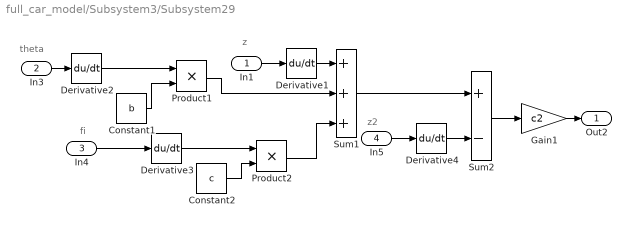
== system full_car_model/Subsystem3/Subsystem29 ==
  note: z
  note: theta
  note: fi
  note: z2
  In1 : Inport  OutDataType=sfix(16)  OutScaling=2^0
  In3 : Inport  Port=2  OutDataType=sfix(16)  OutScaling=2^0
  In4 : Inport  Port=3  OutDataType=sfix(16)  OutScaling=2^0
  In5 : Inport  Port=4  OutDataType=sfix(16)  OutScaling=2^0
  Constant1 : Constant  Value=b  OutDataType=sfix(16)  OutScaling=2^0
  Constant2 : Constant  Value=c  OutDataType=sfix(16)  OutScaling=2^0
  Derivative{1..4} (4 alike) : Derivative
  Gain1 : Gain  Gain=c2  ParameterDataType=sfix(16)  ParameterScaling=2^0  OutDataType=sfix(16)  OutScaling=2^0
  Product1 : Product  OutDataType=sfix(16)  OutScaling=2^0  RndMeth=Zero
  Product2 : Product  OutDataType=sfix(16)  OutScaling=2^0  RndMeth=Zero
  Sum1 : Sum  Inputs=+++  OutDataType=sfix(16)  OutScaling=2^0
  Sum2 : Sum  Inputs=+-  OutDataType=sfix(16)  OutScaling=2^0
  Out2 : Outport  OutDataType=sfix(16)  OutScaling=2^0
  wires:
  Derivative3/1 -> Product2/1
  Derivative2/1 -> Product1/1
  Derivative1/1 -> Sum1/1
  In1/1 -> Derivative1/1
  In3/1 -> Derivative2/1
  In4/1 -> Derivative3/1
  Constant1/1 -> Product1/2
  Product1/1 -> Sum1/2
  Constant2/1 -> Product2/2
  In5/1 -> Derivative4/1
  Product2/1 -> Sum1/3
  Gain1/1 -> Out2/1
  Sum2/1 -> Gain1/1
  Sum1/1 -> Sum2/1
  Derivative4/1 -> Sum2/2

== system full_car_model/Subsystem3/Subsystem30 ==
  note: q2
  note: z2
  In1 : Inport  OutDataType=sfix(16)  OutScaling=2^0
  In5 : Inport  Port=2  OutDataType=sfix(16)  OutScaling=2^0
  Gain1 : Gain  Gain=k02  ParameterDataType=sfix(16)  ParameterScaling=2^0  OutDataType=sfix(16)  OutScaling=2^0
  Sum1 : Sum  Inputs=+-  OutDataType=sfix(16)  OutScaling=2^0
  Out2 : Outport  OutDataType=sfix(16)  OutScaling=2^0
  wires:
  Gain1/1 -> Out2/1
  Sum1/1 -> Gain1/1
  In1/1 -> Sum1/1
  In5/1 -> Sum1/2

== system full_car_model/Subsystem3/Subsystem31 ==
  note: z2
  note: q2
  In1 : Inport  OutDataType=sfix(16)  OutScaling=2^0
  In5 : Inport  Port=2  OutDataType=sfix(16)  OutScaling=2^0
  Derivative : Derivative
  Derivative1 : Derivative
  Gain1 : Gain  Gain=c02  ParameterDataType=sfix(16)  ParameterScaling=2^0  OutDataType=sfix(16)  OutScaling=2^0
  Sum1 : Sum  Inputs=+-  OutDataType=sfix(16)  OutScaling=2^0
  Out2 : Outport  OutDataType=sfix(16)  OutScaling=2^0
  wires:
  In5/1 -> Derivative1/1
  In1/1 -> Derivative/1
  Sum1/1 -> Gain1/1
  Gain1/1 -> Out2/1
  Derivative/1 -> Sum1/1
  Derivative1/1 -> Sum1/2

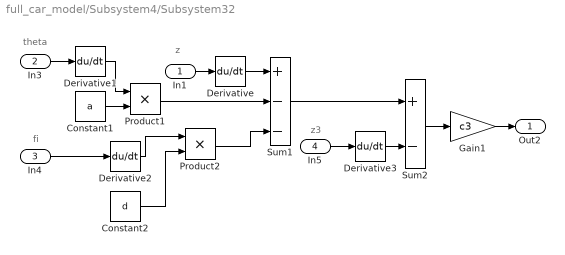
== system full_car_model/Subsystem4/Subsystem32 ==
  note: z3
  note: fi
  note: theta
  note: z
  In1 : Inport  OutDataType=sfix(16)  OutScaling=2^0
  In3 : Inport  Port=2  OutDataType=sfix(16)  OutScaling=2^0
  In4 : Inport  Port=3  OutDataType=sfix(16)  OutScaling=2^0
  In5 : Inport  Port=4  OutDataType=sfix(16)  OutScaling=2^0
  Constant1 : Constant  Value=a  OutDataType=sfix(16)  OutScaling=2^0
  Constant2 : Constant  Value=d  OutDataType=sfix(16)  OutScaling=2^0
  Derivative{,1..3} (4 alike) : Derivative
  Gain1 : Gain  Gain=c3  ParameterDataType=sfix(16)  ParameterScaling=2^0  OutDataType=sfix(16)  OutScaling=2^0
  Product1 : Product  OutDataType=sfix(16)  OutScaling=2^0  RndMeth=Zero
  Product2 : Product  OutDataType=sfix(16)  OutScaling=2^0  RndMeth=Zero
  Sum1 : Sum  Inputs=+--  OutDataType=sfix(16)  OutScaling=2^0
  Sum2 : Sum  Inputs=+-  OutDataType=sfix(16)  OutScaling=2^0
  Out2 : Outport  OutDataType=sfix(16)  OutScaling=2^0
  wires:
  Derivative2/1 -> Product2/1
  Derivative1/1 -> Product1/1
  Derivative/1 -> Sum1/1
  Gain1/1 -> Out2/1
  Product2/1 -> Sum1/3
  In5/1 -> Derivative3/1
  Constant2/1 -> Product2/2
  Product1/1 -> Sum1/2
  Constant1/1 -> Product1/2
  In4/1 -> Derivative2/1
  In3/1 -> Derivative1/1
  In1/1 -> Derivative/1
  Sum1/1 -> Sum2/1
  Derivative3/1 -> Sum2/2
  Sum2/1 -> Gain1/1

== system full_car_model/Subsystem4/Subsystem33 ==
  note: z
  note: theta
  note: fi
  note: z3
  In1 : Inport  OutDataType=sfix(16)  OutScaling=2^0
  In3 : Inport  Port=2  OutDataType=sfix(16)  OutScaling=2^0
  In4 : Inport  Port=3  OutDataType=sfix(16)  OutScaling=2^0
  In5 : Inport  Port=4  OutDataType=sfix(16)  OutScaling=2^0
  Constant1 : Constant  Value=a  OutDataType=sfix(16)  OutScaling=2^0
  Constant2 : Constant  Value=d  OutDataType=sfix(16)  OutScaling=2^0
  Gain1 : Gain  Gain=k3  ParameterDataType=sfix(16)  ParameterScaling=2^0  OutDataType=sfix(16)  OutScaling=2^0
  Product1 : Product  OutDataType=sfix(16)  OutScaling=2^0  RndMeth=Zero
  Product2 : Product  OutDataType=sfix(16)  OutScaling=2^0  RndMeth=Zero
  Sum1 : Sum  Inputs=+--  OutDataType=sfix(16)  OutScaling=2^0
  Sum2 : Sum  Inputs=+-  OutDataType=sfix(16)  OutScaling=2^0
  Out2 : Outport  OutDataType=sfix(16)  OutScaling=2^0
  wires:
  In1/1 -> Sum1/1
  In3/1 -> Product1/1
  In4/1 -> Product2/1
  Constant1/1 -> Product1/2
  Product1/1 -> Sum1/2
  Constant2/1 -> Product2/2
  Product2/1 -> Sum1/3
  Gain1/1 -> Out2/1
  Sum1/1 -> Sum2/1
  Sum2/1 -> Gain1/1
  In5/1 -> Sum2/2

== system full_car_model/Subsystem4/Subsystem34 ==
  note: q3
  note: z3
  In1 : Inport  OutDataType=sfix(16)  OutScaling=2^0
  In5 : Inport  Port=2  OutDataType=sfix(16)  OutScaling=2^0
  Gain1 : Gain  Gain=k03  ParameterDataType=sfix(16)  ParameterScaling=2^0  OutDataType=sfix(16)  OutScaling=2^0
  Sum1 : Sum  Inputs=+-  OutDataType=sfix(16)  OutScaling=2^0
  Out2 : Outport  OutDataType=sfix(16)  OutScaling=2^0
  wires:
  Gain1/1 -> Out2/1
  Sum1/1 -> Gain1/1
  In1/1 -> Sum1/1
  In5/1 -> Sum1/2

== system full_car_model/Subsystem4/Subsystem35 ==
  note: z3
  note: q3
  In1 : Inport  OutDataType=sfix(16)  OutScaling=2^0
  In5 : Inport  Port=2  OutDataType=sfix(16)  OutScaling=2^0
  Derivative : Derivative
  Derivative1 : Derivative
  Gain1 : Gain  Gain=c03  ParameterDataType=sfix(16)  ParameterScaling=2^0  OutDataType=sfix(16)  OutScaling=2^0
  Sum1 : Sum  Inputs=+-  OutDataType=sfix(16)  OutScaling=2^0
  Out2 : Outport  OutDataType=sfix(16)  OutScaling=2^0
  wires:
  In5/1 -> Derivative1/1
  In1/1 -> Derivative/1
  Sum1/1 -> Gain1/1
  Gain1/1 -> Out2/1
  Derivative/1 -> Sum1/1
  Derivative1/1 -> Sum1/2

== system full_car_model/Subsystem5/Subsystem36 ==
  note: z4
  note: fi
  note: theta
  note: z
  In1 : Inport  OutDataType=sfix(16)  OutScaling=2^0
  In3 : Inport  Port=2  OutDataType=sfix(16)  OutScaling=2^0
  In4 : Inport  Port=3  OutDataType=sfix(16)  OutScaling=2^0
  In5 : Inport  Port=4  OutDataType=sfix(16)  OutScaling=2^0
  Constant1 : Constant  Value=b  OutDataType=sfix(16)  OutScaling=2^0
  Constant2 : Constant  Value=d  OutDataType=sfix(16)  OutScaling=2^0
  Gain1 : Gain  Gain=k4  ParameterDataType=sfix(16)  ParameterScaling=2^0  OutDataType=sfix(16)  OutScaling=2^0
  Product1 : Product  OutDataType=sfix(16)  OutScaling=2^0  RndMeth=Zero
  Product2 : Product  OutDataType=sfix(16)  OutScaling=2^0  RndMeth=Zero
  Sum1 : Sum  Inputs=++-  OutDataType=sfix(16)  OutScaling=2^0
  Sum2 : Sum  Inputs=+-  OutDataType=sfix(16)  OutScaling=2^0
  Out2 : Outport  OutDataType=sfix(16)  OutScaling=2^0
  wires:
  Gain1/1 -> Out2/1
  Product2/1 -> Sum1/3
  Constant2/1 -> Product2/2
  Product1/1 -> Sum1/2
  Constant1/1 -> Product1/2
  In4/1 -> Product2/1
  In3/1 -> Product1/1
  In1/1 -> Sum1/1
  Sum1/1 -> Sum2/1
  In5/1 -> Sum2/2
  Sum2/1 -> Gain1/1

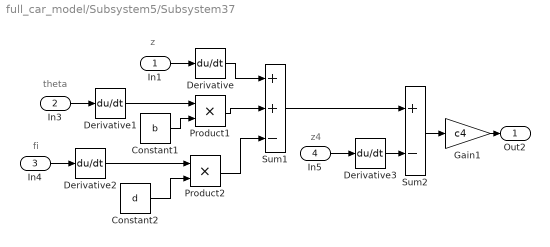
== system full_car_model/Subsystem5/Subsystem37 ==
  note: z
  note: theta
  note: fi
  note: z4
  In1 : Inport  OutDataType=sfix(16)  OutScaling=2^0
  In3 : Inport  Port=2  OutDataType=sfix(16)  OutScaling=2^0
  In4 : Inport  Port=3  OutDataType=sfix(16)  OutScaling=2^0
  In5 : Inport  Port=4  OutDataType=sfix(16)  OutScaling=2^0
  Constant1 : Constant  Value=b  OutDataType=sfix(16)  OutScaling=2^0
  Constant2 : Constant  Value=d  OutDataType=sfix(16)  OutScaling=2^0
  Derivative{,1..3} (4 alike) : Derivative
  Gain1 : Gain  Gain=c4  ParameterDataType=sfix(16)  ParameterScaling=2^0  OutDataType=sfix(16)  OutScaling=2^0
  Product1 : Product  OutDataType=sfix(16)  OutScaling=2^0  RndMeth=Zero
  Product2 : Product  OutDataType=sfix(16)  OutScaling=2^0  RndMeth=Zero
  Sum1 : Sum  Inputs=++-  OutDataType=sfix(16)  OutScaling=2^0
  Sum2 : Sum  Inputs=+-  OutDataType=sfix(16)  OutScaling=2^0
  Out2 : Outport  OutDataType=sfix(16)  OutScaling=2^0
  wires:
  Derivative2/1 -> Product2/1
  Derivative1/1 -> Product1/1
  Derivative/1 -> Sum1/1
  In1/1 -> Derivative/1
  In3/1 -> Derivative1/1
  In4/1 -> Derivative2/1
  Constant1/1 -> Product1/2
  Product1/1 -> Sum1/2
  Constant2/1 -> Product2/2
  In5/1 -> Derivative3/1
  Product2/1 -> Sum1/3
  Gain1/1 -> Out2/1
  Sum1/1 -> Sum2/1
  Sum2/1 -> Gain1/1
  Derivative3/1 -> Sum2/2

== system full_car_model/Subsystem5/Subsystem38 ==
  note: q4
  note: z4
  In1 : Inport  OutDataType=sfix(16)  OutScaling=2^0
  In5 : Inport  Port=2  OutDataType=sfix(16)  OutScaling=2^0
  Gain1 : Gain  Gain=k04  ParameterDataType=sfix(16)  ParameterScaling=2^0  OutDataType=sfix(16)  OutScaling=2^0
  Sum1 : Sum  Inputs=+-  OutDataType=sfix(16)  OutScaling=2^0
  Out2 : Outport  OutDataType=sfix(16)  OutScaling=2^0
  wires:
  Gain1/1 -> Out2/1
  Sum1/1 -> Gain1/1
  In1/1 -> Sum1/1
  In5/1 -> Sum1/2

== system full_car_model/Subsystem5/Subsystem39 ==
  note: z4
  note: q4
  In1 : Inport  OutDataType=sfix(16)  OutScaling=2^0
  In5 : Inport  Port=2  OutDataType=sfix(16)  OutScaling=2^0
  Derivative : Derivative
  Derivative1 : Derivative
  Gain1 : Gain  Gain=c04  ParameterDataType=sfix(16)  ParameterScaling=2^0  OutDataType=sfix(16)  OutScaling=2^0
  Sum1 : Sum  Inputs=+-  OutDataType=sfix(16)  OutScaling=2^0
  Out2 : Outport  OutDataType=sfix(16)  OutScaling=2^0
  wires:
  In5/1 -> Derivative1/1
  In1/1 -> Derivative/1
  Sum1/1 -> Gain1/1
  Gain1/1 -> Out2/1
  Derivative/1 -> Sum1/1
  Derivative1/1 -> Sum1/2

== system full_car_model/Subsystem/Subsystem3/Subsystem8 ==
  note: z1
  note: fi
  note: theta
  note: z
  In1 : Inport  OutDataType=sfix(16)  OutScaling=2^0
  In3 : Inport  Port=2  OutDataType=sfix(16)  OutScaling=2^0
  In4 : Inport  Port=3  OutDataType=sfix(16)  OutScaling=2^0
  In5 : Inport  Port=4  OutDataType=sfix(16)  OutScaling=2^0
  Constant1 : Constant  Value=a  OutDataType=sfix(16)  OutScaling=2^0
  Constant2 : Constant  Value=c  OutDataType=sfix(16)  OutScaling=2^0
  Gain1 : Gain  Gain=k1  ParameterDataType=sfix(16)  ParameterScaling=2^0  OutDataType=sfix(16)  OutScaling=2^0
  Product1 : Product  OutDataType=sfix(16)  OutScaling=2^0  RndMeth=Zero
  Product2 : Product  OutDataType=sfix(16)  OutScaling=2^0  RndMeth=Zero
  Sum1 : Sum  Inputs=+-+  OutDataType=sfix(16)  OutScaling=2^0
  Sum2 : Sum  Inputs=+-  OutDataType=sfix(16)  OutScaling=2^0
  Out2 : Outport  OutDataType=sfix(16)  OutScaling=2^0
  wires:
  Gain1/1 -> Out2/1
  Product2/1 -> Sum1/3
  Constant2/1 -> Product2/2
  Product1/1 -> Sum1/2
  Constant1/1 -> Product1/2
  In4/1 -> Product2/1
  In3/1 -> Product1/1
  In1/1 -> Sum1/1
  Sum1/1 -> Sum2/1
  In5/1 -> Sum2/2
  Sum2/1 -> Gain1/1

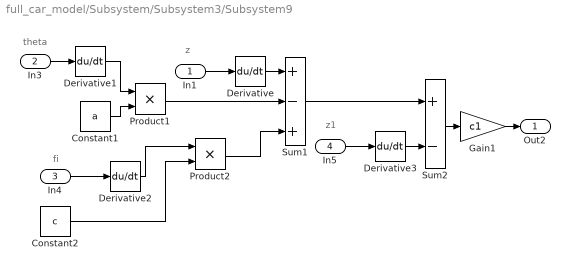
== system full_car_model/Subsystem/Subsystem3/Subsystem9 ==
  note: z
  note: theta
  note: fi
  note: z1
  In1 : Inport  OutDataType=sfix(16)  OutScaling=2^0
  In3 : Inport  Port=2  OutDataType=sfix(16)  OutScaling=2^0
  In4 : Inport  Port=3  OutDataType=sfix(16)  OutScaling=2^0
  In5 : Inport  Port=4  OutDataType=sfix(16)  OutScaling=2^0
  Constant1 : Constant  Value=a  OutDataType=sfix(16)  OutScaling=2^0
  Constant2 : Constant  Value=c  OutDataType=sfix(16)  OutScaling=2^0
  Derivative{,1..3} (4 alike) : Derivative
  Gain1 : Gain  Gain=c1  ParameterDataType=sfix(16)  ParameterScaling=2^0  OutDataType=sfix(16)  OutScaling=2^0
  Product1 : Product  OutDataType=sfix(16)  OutScaling=2^0  RndMeth=Zero
  Product2 : Product  OutDataType=sfix(16)  OutScaling=2^0  RndMeth=Zero
  Sum1 : Sum  Inputs=+-+  OutDataType=sfix(16)  OutScaling=2^0
  Sum2 : Sum  Inputs=+-  OutDataType=sfix(16)  OutScaling=2^0
  Out2 : Outport  OutDataType=sfix(16)  OutScaling=2^0
  wires:
  Derivative2/1 -> Product2/1
  Derivative1/1 -> Product1/1
  Derivative/1 -> Sum1/1
  In1/1 -> Derivative/1
  In3/1 -> Derivative1/1
  In4/1 -> Derivative2/1
  Constant1/1 -> Product1/2
  Product1/1 -> Sum1/2
  Constant2/1 -> Product2/2
  In5/1 -> Derivative3/1
  Product2/1 -> Sum1/3
  Gain1/1 -> Out2/1
  Sum1/1 -> Sum2/1
  Derivative3/1 -> Sum2/2
  Sum2/1 -> Gain1/1

== system full_car_model/Subsystem/Subsystem4/Subsystem10 ==
  note: z2
  note: fi
  note: theta
  note: z
  In1 : Inport  OutDataType=sfix(16)  OutScaling=2^0
  In3 : Inport  Port=2  OutDataType=sfix(16)  OutScaling=2^0
  In4 : Inport  Port=3  OutDataType=sfix(16)  OutScaling=2^0
  In5 : Inport  Port=4  OutDataType=sfix(16)  OutScaling=2^0
  Constant1 : Constant  Value=b  OutDataType=sfix(16)  OutScaling=2^0
  Constant2 : Constant  Value=c  OutDataType=sfix(16)  OutScaling=2^0
  Gain1 : Gain  Gain=k2  ParameterDataType=sfix(16)  ParameterScaling=2^0  OutDataType=sfix(16)  OutScaling=2^0
  Product1 : Product  OutDataType=sfix(16)  OutScaling=2^0  RndMeth=Zero
  Product2 : Product  OutDataType=sfix(16)  OutScaling=2^0  RndMeth=Zero
  Sum1 : Sum  Inputs=+++  OutDataType=sfix(16)  OutScaling=2^0
  Sum2 : Sum  Inputs=+-  OutDataType=sfix(16)  OutScaling=2^0
  Out2 : Outport  OutDataType=sfix(16)  OutScaling=2^0
  wires:
  Gain1/1 -> Out2/1
  Product2/1 -> Sum1/3
  Constant2/1 -> Product2/2
  Product1/1 -> Sum1/2
  Constant1/1 -> Product1/2
  In4/1 -> Product2/1
  In3/1 -> Product1/1
  In1/1 -> Sum1/1
  Sum1/1 -> Sum2/1
  In5/1 -> Sum2/2
  Sum2/1 -> Gain1/1

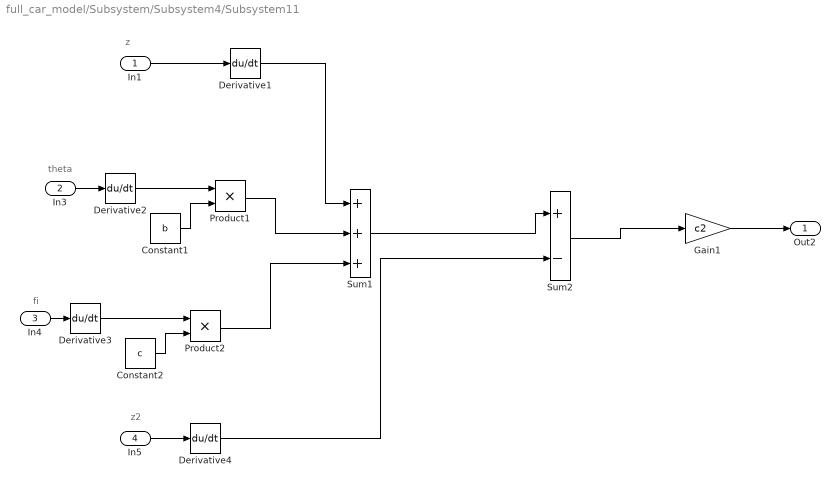
== system full_car_model/Subsystem/Subsystem4/Subsystem11 ==
  note: z
  note: theta
  note: fi
  note: z2
  In1 : Inport  OutDataType=sfix(16)  OutScaling=2^0
  In3 : Inport  Port=2  OutDataType=sfix(16)  OutScaling=2^0
  In4 : Inport  Port=3  OutDataType=sfix(16)  OutScaling=2^0
  In5 : Inport  Port=4  OutDataType=sfix(16)  OutScaling=2^0
  Constant1 : Constant  Value=b  OutDataType=sfix(16)  OutScaling=2^0
  Constant2 : Constant  Value=c  OutDataType=sfix(16)  OutScaling=2^0
  Derivative{1..4} (4 alike) : Derivative
  Gain1 : Gain  Gain=c2  ParameterDataType=sfix(16)  ParameterScaling=2^0  OutDataType=sfix(16)  OutScaling=2^0
  Product1 : Product  OutDataType=sfix(16)  OutScaling=2^0  RndMeth=Zero
  Product2 : Product  OutDataType=sfix(16)  OutScaling=2^0  RndMeth=Zero
  Sum1 : Sum  Inputs=+++  OutDataType=sfix(16)  OutScaling=2^0
  Sum2 : Sum  Inputs=+-  OutDataType=sfix(16)  OutScaling=2^0
  Out2 : Outport  OutDataType=sfix(16)  OutScaling=2^0
  wires:
  Derivative3/1 -> Product2/1
  Derivative2/1 -> Product1/1
  Derivative1/1 -> Sum1/1
  In1/1 -> Derivative1/1
  In3/1 -> Derivative2/1
  In4/1 -> Derivative3/1
  Constant1/1 -> Product1/2
  Product1/1 -> Sum1/2
  Constant2/1 -> Product2/2
  In5/1 -> Derivative4/1
  Product2/1 -> Sum1/3
  Gain1/1 -> Out2/1
  Sum1/1 -> Sum2/1
  Derivative4/1 -> Sum2/2
  Sum2/1 -> Gain1/1

== system full_car_model/Subsystem/Subsystem5/Subsystem12 ==
  note: z
  note: theta
  note: fi
  note: z3
  In1 : Inport  OutDataType=sfix(16)  OutScaling=2^0
  In3 : Inport  Port=2  OutDataType=sfix(16)  OutScaling=2^0
  In4 : Inport  Port=3  OutDataType=sfix(16)  OutScaling=2^0
  In5 : Inport  Port=4  OutDataType=sfix(16)  OutScaling=2^0
  Constant1 : Constant  Value=a  OutDataType=sfix(16)  OutScaling=2^0
  Constant2 : Constant  Value=d  OutDataType=sfix(16)  OutScaling=2^0
  Gain1 : Gain  Gain=k3  ParameterDataType=sfix(16)  ParameterScaling=2^0  OutDataType=sfix(16)  OutScaling=2^0
  Product1 : Product  OutDataType=sfix(16)  OutScaling=2^0  RndMeth=Zero
  Product2 : Product  OutDataType=sfix(16)  OutScaling=2^0  RndMeth=Zero
  Sum1 : Sum  Inputs=+--  OutDataType=sfix(16)  OutScaling=2^0
  Sum2 : Sum  Inputs=+-  OutDataType=sfix(16)  OutScaling=2^0
  Out2 : Outport  OutDataType=sfix(16)  OutScaling=2^0
  wires:
  In1/1 -> Sum1/1
  In3/1 -> Product1/1
  In4/1 -> Product2/1
  Constant1/1 -> Product1/2
  Product1/1 -> Sum1/2
  Constant2/1 -> Product2/2
  Product2/1 -> Sum1/3
  Gain1/1 -> Out2/1
  Sum1/1 -> Sum2/1
  In5/1 -> Sum2/2
  Sum2/1 -> Gain1/1
